simulink model "q3"  (R2018a)
settings: Solver=VariableStepAuto  StartTime=0.0  StopTime=10.0  RelTol=1e-3
settings Model: Creator=hp  LastModifiedBy=hp

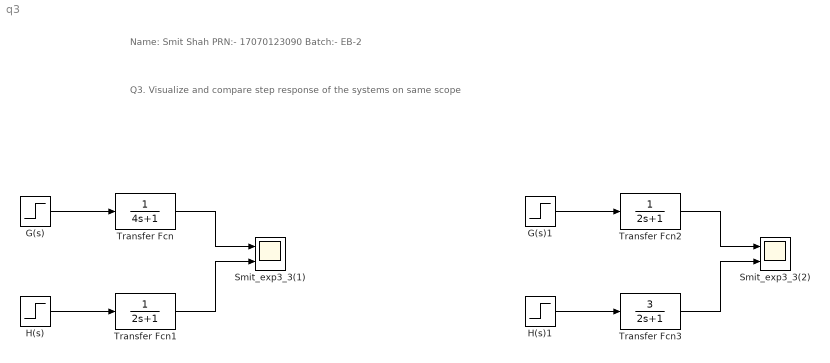
== system q3 ==
  note: Name: Smit Shah PRN:- 17070123090 Batch:- EB-2
  note: Q3. Visualize and compare step response of the systems on same scope
  G(s) : Step  SampleTime=0
  G(s)1 : Step  SampleTime=0
  H(s) : Step  SampleTime=0
  H(s)1 : Step  SampleTime=0
  Smit_exp3_3(1) : Scope  NumInputPorts=2
  Smit_exp3_3(2) : Scope  NumInputPorts=2
  Transfer Fcn : TransferFcn  Denominator=[4 1]
  Transfer Fcn1 : TransferFcn  Denominator=[2 1]
  Transfer Fcn2 : TransferFcn  Denominator=[2 1]
  Transfer Fcn3 : TransferFcn  Numerator=[3]  Denominator=[2 1]
  wires:
  G(s)/1 -> Transfer Fcn/1
  H(s)/1 -> Transfer Fcn1/1
  Transfer Fcn/1 -> Smit_exp3_3(1)/1
  Transfer Fcn1/1 -> Smit_exp3_3(1)/2
  Transfer Fcn2/1 -> Smit_exp3_3(2)/1
  Transfer Fcn3/1 -> Smit_exp3_3(2)/2
  H(s)1/1 -> Transfer Fcn3/1
  G(s)1/1 -> Transfer Fcn2/1
